simulink model "gNautilus_REC"  (R2017b)
settings: Solver=FixedStepDiscrete  StartTime=0.0  StopTime=180  RelTol=1e-3  EnableMultiTasking=on
model workspace (MAT data in the model file):
  cfg_native : struct (value not decoded)
  en_add_channels = 127
  host_ip = 2130706433
  host_port = 50223
  local_ip = 2130706433
  local_port = 50224
  num_en_channels = 8
  num_samples = 4
  sample_rate = 250
  serial_number = 'NB-2016.09.83'
undefined symbols (not defined in the file): NB
libraries: gNautilusLib x1, gNautilusTools x1, gtecHighspeedLib x1
settings Model: Creator=g.tec Maresch  LastModifiedBy=Gabriel
settings DataIOCC: LimitDataPoints=on  SaveFormat=Array  SignalLoggingSaveFormat=ModelDataLogs
settings OptimizationCC: ExpressionDepthLimit=2147483647  LifeSpan=inf
settings DebuggingCC: UnderspecifiedInitializationDetection=Classic  MergeDetectMultiDrivingBlocksExec=none  SolverPrmCheckMsg=warning  FcnCallInpInsideContextMsg=warning  FrameProcessingCompatibilityMsg=none  StateNameClashWarn=warning  SFUnexpectedBacktrackingDiag=warning  SFNoUnconditionalDefaultTransitionDiag=warning  SFExecutionAtInitializationDiag=none
settings HardwareCC: ProdBitPerPointer=32  ProdBitPerSizeT=32  ProdBitPerPtrDiffT=32  ProdLargestAtomicFloat=None  ProdIntDivRoundTo=Undefined  ProdEndianess=Unspecified  ProdWordSize=32  ProdHWDeviceType=32-bit Generic
settings ModelReferenceCC: PropagateSignalLabelsOutOfModel=off
settings CodeAppCC: StateflowObjectComments=on
settings GRTTargetCC: TargetLangStandard=C89/C90 (ANSI)  GeneratePreprocessorConditionals=Disable all  CombineOutputUpdateFcns=off  GRTInterface=on
settings ConfigComp: CovMetricSettings=dw  CovHtmlReporting=on  CovSaveCumulativeToWorkspaceVar=on  CovSaveSingleToWorkspaceVar=on  CovExternalEMLEnable=off

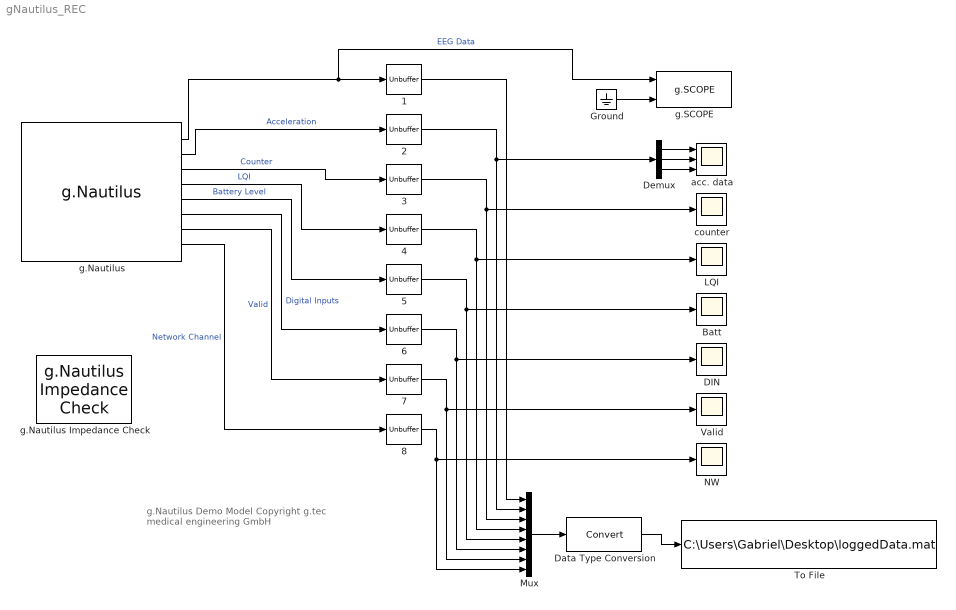
== system gNautilus_REC ==
  note: g.Nautilus Demo Model
      | Copyright g.tec medical engineering GmbH
  {1..8} (8 alike) : Unbuffer
  Batt : Scope
  DIN : Scope
  Data Type Conversion : DataTypeConversion
  Demux : Demux  Outputs=3
  Ground : Ground
  LQI : Scope
  Mux : Mux  Inputs=8
  NW : Scope
  To File : ToFile  Filename=C:\Users\Gabriel\Desktop\loggedData.mat  MatrixName=y
  Valid : Scope
  acc. data : Scope  NumInputPorts=3
  counter : Scope
  g.Nautilus : gNautilusLib/g.Nautilus  Tag=g.Nautilus  Description=Operates a g.Nautilus device and provides acquired data on its outputs.  sample_rate=250  local_ip=2130706433  local_port=50224  host_ip=2130706433  host_port=50223  serial_number=NB-2016.09.83  num_samples=4  num_en_channels=8  add_channels=127
      settings: SourceProductName=g.Nautilus
  g.Nautilus Impedance Check : gNautilusTools/g.Nautilus Impedance Check
  g.SCOPE : gtecHighspeedLib/g.SCOPE
      settings: SourceProductName=g.tec Highspeed Library
  wires:
  2/1 -> Demux/1, Mux/2
  3/1 -> counter/1, Mux/3
  4/1 -> LQI/1, Mux/4
  g.Nautilus/1 -> g.SCOPE/1, 1/1  "EEG Data"
  g.Nautilus/2 -> 2/1  "Acceleration"
  g.Nautilus/3 -> 3/1  "Counter"
  g.Nautilus/4 -> 4/1  "LQI"
  Demux/1 -> acc. data/1
  Demux/2 -> acc. data/2
  Demux/3 -> acc. data/3
  5/1 -> Batt/1, Mux/5
  g.Nautilus/5 -> 5/1  "Battery Level"
  6/1 -> DIN/1, Mux/6
  g.Nautilus/6 -> 6/1  "Digital Inputs"
  7/1 -> Valid/1, Mux/7
  8/1 -> NW/1, Mux/8
  g.Nautilus/7 -> 7/1  "Valid"
  g.Nautilus/8 -> 8/1  "Network Channel"
  Data Type Conversion/1 -> To File/1
  Mux/1 -> Data Type Conversion/1
  1/1 -> Mux/1
  Ground/1 -> g.SCOPE/2
